simulink model "UDPLink_Distal"  (R2020a)
settings: Solver=FixedStepAuto  StartTime=0.0  StopTime=inf  RelTol=1e-3  EnableMultiTasking=on
undefined symbols (not defined in the file or in its folder): IO392, IO397
libraries: xpcutilitieslib x9, hdlsllib x5, slrtlib x3, speedgoatlib_fpga_quadrature x2, speedgoatlib_fpga x2, xpcrtudplib x2, speedgoatlib_fpga_analog_io x1
settings Model: SimulationMode=external  Creator=ViconLab  LastModifiedBy=ViconLab
settings SolverCC: ConcurrentTasks=on  AutoInsertRateTranBlk=on
settings DataIOCC: SaveFormat=StructureWithTime
settings OptimizationCC: BlockReduction=off  OptimizeBlockIOStorage=off
settings HardwareCC: ProdBitPerPointer=32  ProdBitPerSizeT=32  ProdBitPerPtrDiffT=32  ProdLargestAtomicFloat=None  ProdWordSize=32  ProdLongLongMode=on  ProdHWDeviceType=Generic->32-bit x86 compatible
settings RTWCC: Description=Simulink Real-Time  SystemTargetFile=slrt.tlc  TemplateMakefile=slrt_default_tmf  CodeExecutionProfiling=on  RTWCompilerOptimization=on
settings SimulinkRealTimeCC: SupportVariableSizeSignals=on  RL32LogTETModifier=off  xPCConcurrentTasks=on

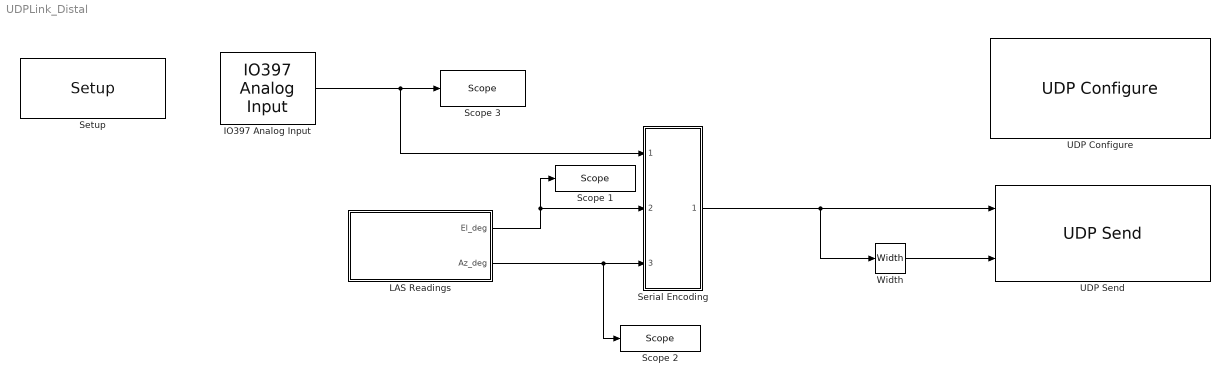
== system UDPLink_Distal ==
  IO397 Analog Input : speedgoatlib_fpga_analog_io/IO397 Analog Input  id=2  chan=1  range=+10 V  trigger=Initiator  ts=-1  pciSlot=-1  board=IO397-50k
      settings: SourceProductName=Simulink Real-Time: Speedgoat I/O Driver Library
  "LAS Readings " : Subsystem
  Scope 1 : slrtlib/Displays and Logging/Scope   scopeno=1  scopetype=Target  autostart=on  viewmode=Graphical sliding  formatstr='%15.6f'  grid=on  ylimits=[0,8000]  nosamples=500  noprepostsamples=0  interleave=1  triggermode=FreeRun  triggersignal=1  trigsignalfromport=off  triggerlevel=0.0  triggerslope=Either  triggerscope=1  triggersample=0  filename=data.dat  mode=Lazy  writesize=512  autorestart=off  dynamicfilemode=off  maxwritefilesize=512*1024^2
  Scope 2 : slrtlib/Displays and Logging/Scope   scopeno=2  scopetype=Target  autostart=on  viewmode=Graphical sliding  formatstr='%15.6f'  grid=on  ylimits=[0,8000]  nosamples=500  noprepostsamples=0  interleave=1  triggermode=FreeRun  triggersignal=1  trigsignalfromport=off  triggerlevel=0.0  triggerslope=Either  triggerscope=1  triggersample=0  filename=data.dat  mode=Lazy  writesize=512  autorestart=off  dynamicfilemode=off  maxwritefilesize=512*1024^2
  Scope 3 : slrtlib/Displays and Logging/Scope   scopeno=3  scopetype=Target  autostart=on  viewmode=Numerical  formatstr='%15.6f'  grid=on  ylimits=[0,0]  nosamples=2000  noprepostsamples=0  interleave=1  triggermode=FreeRun  triggersignal=1  trigsignalfromport=off  triggerlevel=0.0  triggerslope=Either  triggerscope=1  triggersample=0  filename=data.dat  mode=Lazy  writesize=512  autorestart=off  dynamicfilemode=off  maxwritefilesize=512*1024^2
  Serial Encoding : Subsystem
  Setup : speedgoatlib_fpga/Setup/Setup  board=IO397-50k  id=2  device_id=1  frontIO=None  rearIO=None  bitstreamFile=speedgoat_IO397_50k_CI_02113.mat  rev=1.0  timestamp_string=21/04/20 11:41:53  fpgaFreq=75 MHz  fpgaTick=13.33 ns  ProgSpiFlash=off  ProgBPIFlash=off  pciSlot=-1  PullRPort0=pull-up 3.3V  VioPort0=3.3V  PullRPort1=pull-up 3.3V  VioPort1=3.3V  PullRPort2=pull-up 3.3V  VioPort2=3.3V  PullRPort3=pull-up 3.3V  VioPort3=3.3V  PullRPort4=pull-up 3.3V  VioPort4=3.3V  PullRPort5=pull-up 3.3V  VioPort5=3.3V  PullRPort6=pull-up 3.3V  VioPort6=3.3V  PullRPort15=pull-up 3.3V  PullRPort31=pull-up 3.3V  PullRPort47=pull-up 3.3V  PullRPort63=pull-up 3.3V
      settings: SourceProductName=Simulink Real-Time: Speedgoat Library
  UDP Configure : xpcrtudplib/UDP Configure  Priority=-1  IpAddress=30.30.30.2  SubnetMask=255.255.255.0  Gateway=0.0.0.0  PciBus=13  PciSlot=0  PciFunction=0  ID=1  tune=0  disable=off  enableMulticast=off  MulticastIpAddress={}  MulticastMask={}
      settings: SourceProductBaseCode=XP
  UDP Send : xpcrtudplib/UDP Send  ipAddressVal=30.30.30.2  localPort=-1  toAddress=30.30.30.1  toPort=25001  sampleTime=1e-3
      settings: SourceProductBaseCode=XP
  Width : Width
  wires:
  "LAS Readings "/1(El_deg) -> Serial Encoding/2("Serial_El "), Scope 1/1
  Serial Encoding/1(Out1) -> Width/1, UDP Send/1
  "LAS Readings "/2(Az_deg) -> Serial Encoding/3(Serial_Az), Scope 2/1
  Width/1 -> UDP Send/2
  IO397 Analog Input/1 -> Serial Encoding/1(Serial_Lc), Scope 3/1

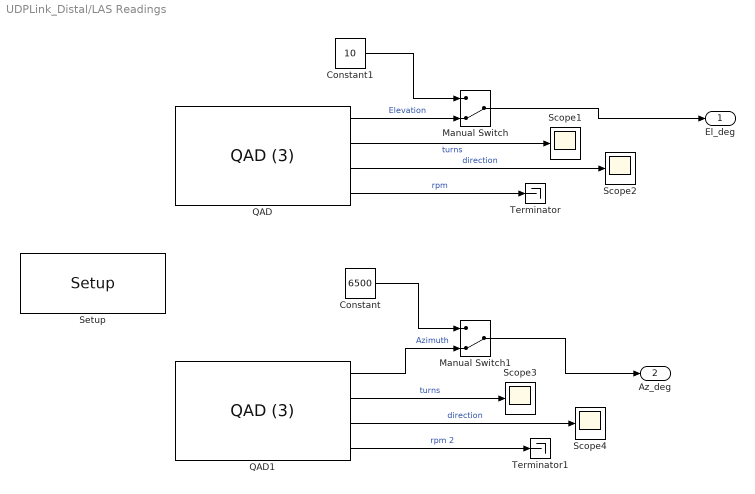
== system UDPLink_Distal/LAS Readings  ==
  Constant : Constant  Value=6500
  Constant1 : Constant  Value=10
  Manual Switch : ManualSwitch  CurrentSetting=0
  Manual Switch1 : ManualSwitch  CurrentSetting=0
  QAD : speedgoatlib_fpga_quadrature/QAD (3)  id=1  board=IO392-50k  chan=[2]  resetOnStart=on  ts=1e-3  pciSlot=-1  operatingMode=Quadrature decoder  indexControlMode=Reset on index  resolution=4x  stepsPerRevolution=[8191]  latchMode=Disabled  interpolatePosition=off  invertAB=off  showClearPositionInput=off  showClearIndexFoundInput=off  showPositionOutput=on  showTurnOutput=on  showSpeedOutput=on  showDirectionOutput=on  showIndexFoundOutput=off
      settings: SourceProductName=Simulink Real-Time: Speedgoat I/O Driver Library
  QAD1 : speedgoatlib_fpga_quadrature/QAD (3)  id=1  board=IO392-50k  chan=[1]  resetOnStart=on  ts=1e-3  pciSlot=-1  operatingMode=Quadrature decoder  indexControlMode=Reset on index  resolution=4x  stepsPerRevolution=[8191]  latchMode=Disabled  interpolatePosition=off  invertAB=off  showClearPositionInput=off  showClearIndexFoundInput=off  showPositionOutput=on  showTurnOutput=on  showSpeedOutput=on  showDirectionOutput=on  showIndexFoundOutput=off
      settings: SourceProductName=Simulink Real-Time: Speedgoat I/O Driver Library
  Scope{1..4} (4 alike) : Scope
  Setup : speedgoatlib_fpga/Setup/Setup  board=IO392-50k  id=1  device_id=1  frontIO=None  rearIO=None  bitstreamFile=speedgoat_IO392_50k_CI_02244.mat  rev=1.0  timestamp_string=07/12/20 12:10:05  fpgaFreq=75 MHz  fpgaTick=13.33 ns  ProgSpiFlash=off  ProgBPIFlash=off  pciSlot=-1  PullRPort0=pull-up 3.3V  VioPort0=3.3V  PullRPort1=pull-up 3.3V  VioPort1=3.3V  PullRPort2=pull-up 3.3V  VioPort2=3.3V  PullRPort3=pull-up 3.3V  VioPort3=3.3V  PullRPort4=pull-up 3.3V  VioPort4=3.3V  PullRPort5=pull-up 3.3V  VioPort5=3.3V  PullRPort6=pull-up 3.3V  VioPort6=3.3V  PullRPort15=pull-up 3.3V  PullRPort31=pull-up 3.3V  PullRPort47=pull-up 3.3V  PullRPort63=pull-up 3.3V
      settings: SourceProductName=Simulink Real-Time: Speedgoat Library
  Terminator : Terminator
  Terminator1 : Terminator
  El_deg : Outport
  Az_deg : Outport  Port=2
  wires:
  QAD1/2 -> Scope3/1  "turns"
  QAD/3 -> Scope2/1  "direction"
  QAD/4 -> Terminator/1  "rpm"
  QAD1/3 -> Scope4/1  "direction"
  QAD/2 -> Scope1/1  "turns"
  QAD1/4 -> Terminator1/1  "rpm 2"
  QAD/1 -> Manual Switch/2  "Elevation"
  Manual Switch/1 -> El_deg/1
  QAD1/1 -> Manual Switch1/2  "Azimuth"
  Manual Switch1/1 -> Az_deg/1
  Constant/1 -> Manual Switch1/1
  Constant1/1 -> Manual Switch/1

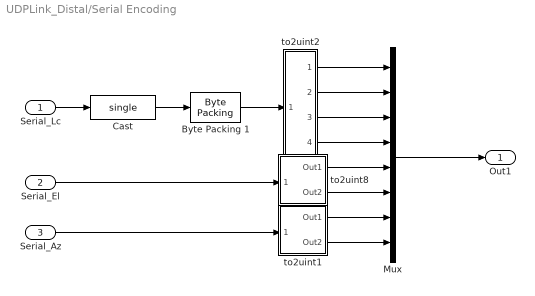
== system UDPLink_Distal/Serial Encoding ==
  Serial_Lc : Inport
  "Serial_El " : Inport  Port=2
  Serial_Az : Inport  Port=3
  Byte Packing 1 : xpcutilitieslib/Byte Packing   MaskPackedDataType=uint32  MaskUnpackedDataTypes={'single'}  MaskAlignment=1
  Cast : DataTypeConversion  OutDataTypeStr=single
  Mux : Mux  Inputs=8
  to2uint1 : Subsystem
  to2uint2 : Subsystem
  to2uint8 : Subsystem
  Out1 : Outport
  wires:
  "Serial_El "/1 -> to2uint8/1(" ")
  Serial_Az/1 -> to2uint1/1(" ")
  to2uint2/3(Out1) -> Mux/3
  to2uint2/4(Out2) -> Mux/4
  to2uint8/1(Out1) -> Mux/5
  to2uint8/2(Out2) -> Mux/6
  to2uint1/1(Out1) -> Mux/7
  to2uint1/2(Out2) -> Mux/8
  Mux/1 -> Out1/1
  Byte Packing 1/1 -> to2uint2/1(" ")
  Cast/1 -> Byte Packing 1/1
  Serial_Lc/1 -> Cast/1
  to2uint2/2(Out3) -> Mux/2
  to2uint2/1(Out4) -> Mux/1

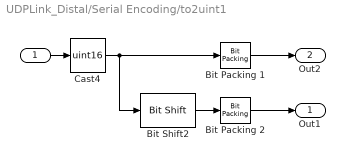
== system UDPLink_Distal/Serial Encoding/to2uint1 ==
  " " : Inport
  Bit Packing 1 : xpcutilitieslib/Bit Packing   MaskBitPatterns={[0:7]}  MaskPackDataType=uint8  MaskPackDataSize=[1]
      settings: SourceProductBaseCode=XP
  Bit Packing 2 : xpcutilitieslib/Bit Packing   MaskBitPatterns={[0:7]}  MaskPackDataType=uint8  MaskPackDataSize=[1]
      settings: SourceProductBaseCode=XP
  Bit Shift2 : hdlsllib/Logic and Bit Operations/Bit Shift  mode=Shift Right Arithmetic  N=8
  Cast4 : DataTypeConversion  OutDataTypeStr=uint16
  Out1 : Outport
  Out2 : Outport  Port=2
  wires:
  " "/1 -> Cast4/1
  Cast4/1 -> Bit Packing 1/1, Bit Shift2/1
  Bit Shift2/1 -> Bit Packing 2/1
  Bit Packing 2/1 -> Out1/1
  Bit Packing 1/1 -> Out2/1

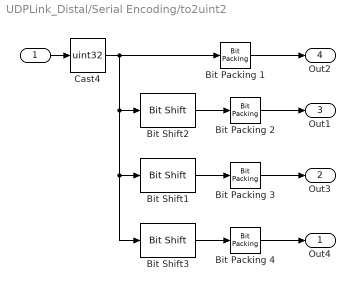
== system UDPLink_Distal/Serial Encoding/to2uint2 ==
  " " : Inport
  Bit Packing {1..4} (4 alike) : xpcutilitieslib/Bit Packing   MaskBitPatterns={[0:7]}  MaskPackDataType=uint8  MaskPackDataSize=[1]
      settings: SourceProductBaseCode=XP
  Bit Shift1 : hdlsllib/Logic and Bit Operations/Bit Shift  mode=Shift Right Arithmetic  N=16
  Bit Shift2 : hdlsllib/Logic and Bit Operations/Bit Shift  mode=Shift Right Arithmetic  N=8
  Bit Shift3 : hdlsllib/Logic and Bit Operations/Bit Shift  mode=Shift Right Arithmetic  N=24
  Cast4 : DataTypeConversion  OutDataTypeStr=uint32
  Out4 : Outport
  Out3 : Outport  Port=2
  Out1 : Outport  Port=3
  Out2 : Outport  Port=4
  wires:
  " "/1 -> Cast4/1
  Cast4/1 -> Bit Packing 1/1, Bit Shift1/1, Bit Shift3/1, Bit Shift2/1
  Bit Shift2/1 -> Bit Packing 2/1
  Bit Packing 2/1 -> Out1/1
  Bit Packing 1/1 -> Out2/1
  Bit Packing 3/1 -> Out3/1
  Bit Shift1/1 -> Bit Packing 3/1
  Bit Shift3/1 -> Bit Packing 4/1
  Bit Packing 4/1 -> Out4/1

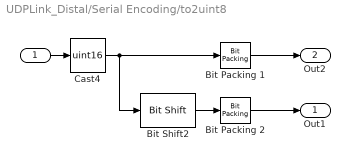
== system UDPLink_Distal/Serial Encoding/to2uint8 ==
  " " : Inport
  Bit Packing 1 : xpcutilitieslib/Bit Packing   MaskBitPatterns={[0:7]}  MaskPackDataType=uint8  MaskPackDataSize=[1]
      settings: SourceProductBaseCode=XP
  Bit Packing 2 : xpcutilitieslib/Bit Packing   MaskBitPatterns={[0:7]}  MaskPackDataType=uint8  MaskPackDataSize=[1]
      settings: SourceProductBaseCode=XP
  Bit Shift2 : hdlsllib/Logic and Bit Operations/Bit Shift  mode=Shift Right Arithmetic  N=8
  Cast4 : DataTypeConversion  OutDataTypeStr=uint16
  Out1 : Outport
  Out2 : Outport  Port=2
  wires:
  Bit Shift2/1 -> Bit Packing 2/1
  Cast4/1 -> Bit Shift2/1, Bit Packing 1/1
  " "/1 -> Cast4/1
  Bit Packing 2/1 -> Out1/1
  Bit Packing 1/1 -> Out2/1
